simulink model "closedlooptemplate"  (R2024a)
settings: Solver=VariableStepAuto  StartTime=0.0  StopTime=10.0  RelTol=1e-3
values from neighbouring files (symbols this model uses):
  A_air = 0.00588710854841    [run1.mat]    (also in run2.mat)
  Cs = 0.9    [run1.mat]    (also in run2.mat)
  h = 0.0127000254001    [run1.mat]    (also in run2.mat)
  m = 100    [run1.mat]    (also in run2.mat)
  T_f = 21    [run1.mat]    (also in run2.mat)
libraries: slctrl_linear x2, slpidlib x1
settings Model: Creator=veswaranandam  LastModifiedBy=veswaranandam

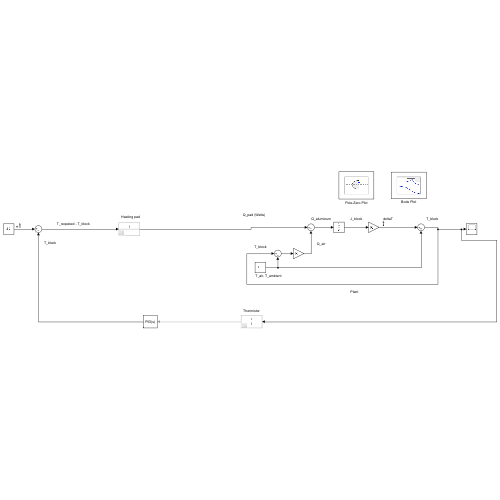
[thumbnail: Simulink's stored preview of the top-level diagram]
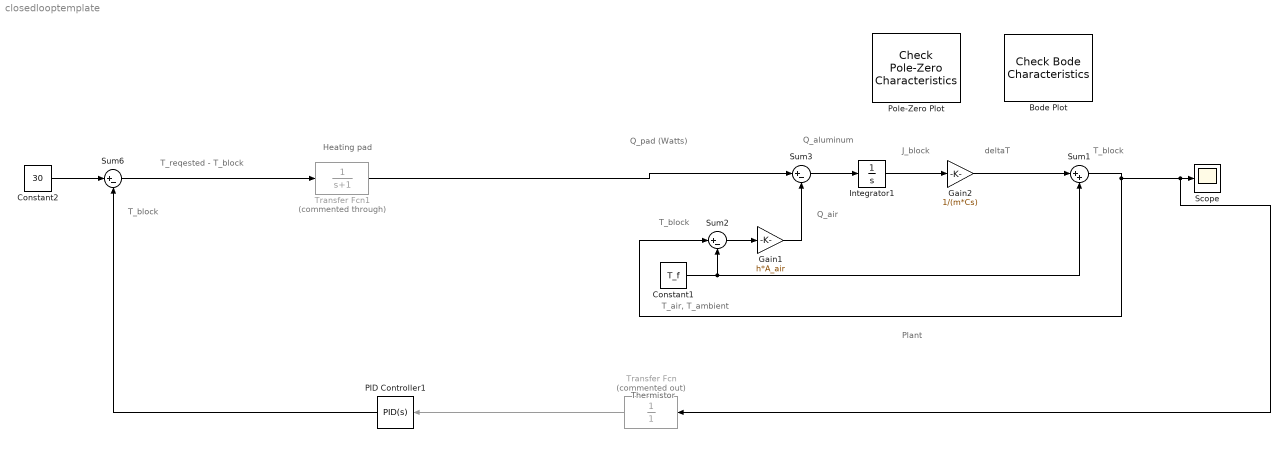
== system closedlooptemplate ==
  note: Plant
  note: Thermistor
  note: Heating pad
  note: T_air, T_ambient
  note: T_block
  note: deltaT
  note: J_block
  note: Q_aluminum
  note: Q_pad (Watts)
  note: T_block
  note: Q_air
  note: T_block
  note: T_reqested - T_block
  Bode Plot : slctrl_linear/Check Bode  Characteristics  InstantiateOnLoad=on  SaveOperatingPoints=off  LinearizationIOs={'/Constant2', 1, 'in', 'off', '';'/Gain2', 1, 'out', 'off', ''}  LinearizeAt=SnapshotTimes  SnapshotTimes=[0]  TriggerType=rising  SampleTime=auto  RateConversionMethod=zoh  PreWarpFreq=10  UseExactDelayModel=off  UseFullBlockNameLabels=off  UseBusSignalLabels=off  enabled=on  stopWhenAssertionFail=off  export=off  ViewDlgPos=[1 41 768 748.8]  OpenViewOnLoad=off  LaunchViewOnOpen=off  FrequencyUnits=rad/s  MagnitudeUnits=dB  PhaseUnits=deg  TimeUnits=seconds  EnableUpperBound=off  UpperBoundFrequencies=[]  UpperBoundMagnitudes=[]  EnableLowerBound=off  LowerBoundFrequencies=[]  LowerBoundMagnitudes=[]
      settings: LibrarySourceBlock=slctrlblks/Linear Analysis Plots/Bode Plot  SaveToWorkspace=off  SaveName=sys
  Constant1 : Constant  Value=T_f
  Constant2 : Constant  Value=30
  Gain1 : Gain  Gain=h*A_air
  Gain2 : Gain  Gain=1/(m*Cs)
  Integrator1 : Integrator
  PID Controller1 : slpidlib/PID Controller  Controller=PID  Form=Parallel  TimeDomain=Continuous-time  UseExternalTs=off  SampleTime=-1  IntegratorMethod=Forward Euler  FilterMethod=Forward Euler  ControllerParametersSource=internal  P=1  I=1  UseKiTs=off  D=0  UseExternalDerivativeSource=off  N=100  UseFilter=on  TunerSelectOption=Transfer Function Based (PID Tuner App)  InitialConditionSource=internal  InitialConditionForIntegrator=0  InitialConditionForFilter=0  DifferentiatorICPrevScaledInput=0  ExternalReset=none  TrackingMode=off  Kt=1  LimitOutput=off  SatLimitsSource=internal  UpperSaturationLimit=inf  LowerSaturationLimit=-inf  LinearizeAsGain=on  AntiWindupMode=none  Kb=1  LimitIntegrator=off  UpperIntegratorSaturationLimit=inf  LowerIntegratorSaturationLimit=-inf  POutMin=[]  POutMax=[]  IOutMin=[]  IOutMax=[]  DOutMin=[]  DOutMax=[]  NOutMin=[]  NOutMax=[]  SumOutMin=[]  SumOutMax=[]  SaturationOutMin=[]  SaturationOutMax=[]  PParamMin=[]  PParamMax=[]  IParamMin=[]  IParamMax=[]  DParamMin=[]  DParamMax=[]  NParamMin=[]  NParamMax=[]  KbParamMin=[]  KbParamMax=[]  KtParamMin=[]  KtParamMax=[]  KbOutMin=[]  KbOutMax=[]  KtOutMin=[]  KtOutMax=[]  IntegratorOutMin=[]  IntegratorOutMax=[]  FilterOutMin=[]  FilterOutMax=[]  SumI1OutMin=[]  SumI1OutMax=[]  SumI2OutMin=[]  SumI2OutMax=[]  SumI3OutMin=[]  SumI3OutMax=[]  SumI4OutMin=[]  SumI4OutMax=[]  SumDOutMin=[]  SumDOutMax=[]  DifferentiatorOutMin=[]  DifferentiatorOutMax=[]  FilterDiffOutCoefMin=[]  FilterDiffOutCoefMax=[]  ReciprocalOutMin=[]  ReciprocalOutMax=[]  SumDenOutMin=[]  SumDenOutMax=[]  SumNumOutMin=[]  SumNumOutMax=[]  DivideOutMin=[]  DivideOutMax=[]  UdiffTsProdOutMin=[]  UdiffTsProdOutMax=[]  NTsProdOutMin=[]  NTsProdOutMax=[]  UintegralTsProdOutMin=[]  UintegralTsProdOutMax=[]  UngainTsProdOutMin=[]  UngainTsProdOutMax=[]  ClampingZeroOutDataTypeStr=Inherit: Inherit via back propagation  ClampingZeroOutMin=[]  ClampingZeroOutMax=[]  FilterDenConstantOutDataTypeStr=Inherit: Inherit via back propagation  FilterDenConstantOutMin=[]  FilterDenConstantOutMax=[]  PCopyOutDataTypeStr=Inherit: Inherit via back propagation  PCopyOutMin=[]  PCopyOutMax=[]  NCopyOutDataTypeStr=Inherit: Inherit via back propagation  NCopyOutMin=[]  NCopyOutMax=[]  IntegratorContinuousStateAttributes=''  IntegratorStateMustResolveToSignalObject=off  IntegratorRTWStateStorageClass=Auto  FilterContinuousStateAttributes=''  FilterStateMustResolveToSignalObject=off  FilterRTWStateStorageClass=Auto  ParallelPVariant=InternalParameters  IdealPVariant=Disabled  IVariant=InternalParameters  DVariant=InternalParameters  IntegratorVariant=Continuous  SatVariant=Disabled  AWVariant=Passthrough  PCopyVariant=Disabled  TRVariant=Disabled  FdbkBlocksVariant=Forward  IdealPFdbkVariant=Disabled  SatFdbkVariant=Disabled  DerivativeFilterVariant=ContFilter  NVariant=InternalParameters  NCopyVariant=Disabled  FilterICVariant=InternalICsFilter  IntegratorICVariant=InternalICs  ExternalResetVariant=Disabled  TRSumVariant=Passthrough  SumFdbkVariant=Disabled  SumVariant=Sum_PID  TsampFilterVariant=InternalTs  TsampNgainVariant=Passthrough  TsampIntegralVariant=Disabled_SignalSpec  ExternalSaturationOutDataTypeStr=Inherit: Same as second input  DerivativeSourceVariant=ErrorSignal
  Pole-Zero Plot : slctrl_linear/Check Pole-Zero Characteristics  InstantiateOnLoad=on  SaveOperatingPoints=off  LinearizationIOs={'/Constant2', 1, 'in', 'off', '';'/Gain2', 1, 'out', 'off', ''}  LinearizeAt=SnapshotTimes  SnapshotTimes=[0]  TriggerType=rising  SampleTime=auto  RateConversionMethod=zoh  PreWarpFreq=10  UseExactDelayModel=off  UseFullBlockNameLabels=off  UseBusSignalLabels=off  enabled=on  stopWhenAssertionFail=off  export=off  ViewDlgPos=[100 200 510 390]  LaunchViewOnOpen=off  OpenViewOnLoad=on  FrequencyUnits=rad/s  MagnitudeUnits=dB  PhaseUnits=deg  TimeUnits=seconds  EnableSettlingTime=off  SettlingTime=[]  EnablePercentOvershoot=off  PercentOvershoot=[]  EnableDampingRatio=off  DampingRatio=[]  EnableNaturalFrequency=off  NaturalFrequencyBound=>=  NaturalFrequency=[]
      settings: LibrarySourceBlock=slctrlblks/Linear Analysis Plots/Pole-Zero Plot  SaveToWorkspace=off  SaveName=sys
  Scope : Scope
  Sum1 : Sum  Inputs=|++
  Sum2 : Sum  Inputs=|+-
  Sum3 : Sum  Inputs=|+-
  Sum6 : Sum  Inputs=|+-
  Transfer Fcn : TransferFcn  Commented=on  Denominator=[1]
  Transfer Fcn1 : TransferFcn  Commented=through  Denominator=[1 1]
  wires:
  Gain1/1 -> Sum3/2
  Sum2/1 -> Gain1/1
  Constant1/1 -> Sum1/2, Sum2/2
  Transfer Fcn1/1 -> Sum3/1
  Sum3/1 -> Integrator1/1
  Integrator1/1 -> Gain2/1
  Gain2/1 -> Sum1/1
  Sum1/1 -> Transfer Fcn/1, Scope/1, Sum2/1
  Sum6/1 -> Transfer Fcn1/1
  Constant2/1 -> Sum6/1
  Transfer Fcn/1 -> PID Controller1/1
  PID Controller1/1 -> Sum6/2
